simulink model "P1"  (R2023b)
settings: Solver=VariableStepAuto  StartTime=0.0  StopTime=10  RelTol=1e-3
settings Model: Creator=Usuario_UMA  LastModifiedBy=javie

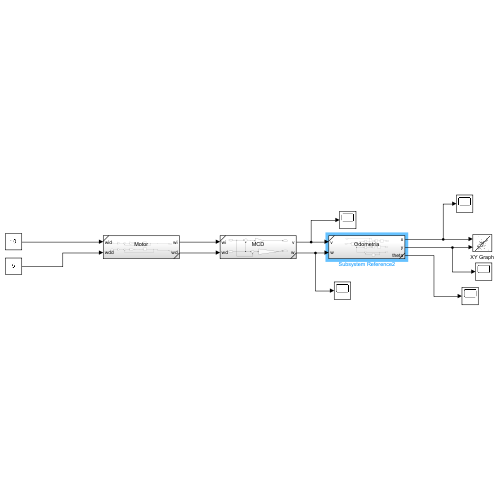
[thumbnail: Simulink's stored preview of the top-level diagram]
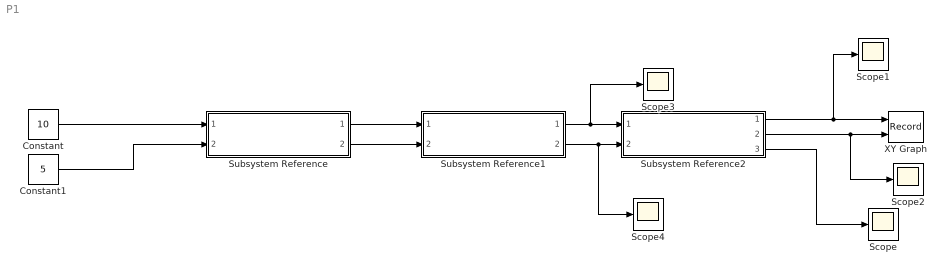
== system P1 ==
  Constant : Constant  Value=10
  Constant1 : Constant  Value=5
  Scope{,1..4} (5 alike) : Scope
  Subsystem Reference : Subsystem  ReferencedSubsystem=Motor
  Subsystem Reference1 : Subsystem  ReferencedSubsystem=MCD
  Subsystem Reference2 : Subsystem  ReferencedSubsystem=Odometria
  XY Graph : Record  FileSettingsInternal="{\"entries\":[{\"content\":{\"excelSettings\":{\"content\":{},\"type\":\"Streamout.ExcelSettings\"}},\"type\":\"Streamout.FileSettingStorage\",\"uuid\":\"\"}],\"packageUris\":[\"http:\\/\\/schema.mathworks.com\\/mf0\\/streamout_blocks\\/R2020a\"],\"version\":\"1.0\"}"  Layout=[1 1]  SignalsInternal="{\"entries\":[{\"content\":{\"signals\":[{\"content\":{\"blockPath\":[],\"dimensions\":[1],\"domain\":\"\",\"lineColor\":\"#a2142f\",\"plots\":[ 1 ],\"port\":1,\"signalID\":1,\"signalName\":\"Subsystem Reference2:1\"},\"type\":\"RecordBlkView.Signal\",\"uuid\":\"\"},{\"content\":{\"blockPath\":[],\"dimensions\":[1],\"domain\":\"\",\"lineColor\":\"#139fff\",\"plots\":[ 1 ],\"port\":2,\"signalID\":2,\"signalName\":\"Subsystem Reference2:2\"},\"type\":\"RecordBlkView.Signal\",\"uuid\":\"\"}]},\"type\":\"RecordBlkView.InputSignals\",\"uuid\":\"\"}],\"packageUris\":[\"http:\\/\\/schema.mathworks.com\\/mf0\\/streamout_blocks\\/R2020a\"],\"version\":\"1.0\"}"  VisualizationBindings="{\"xyplotplugin\":{\"info\":[{\"series\":[{\"bindingParametersList\":[{\"parameter\":\"X-Axis\",\"signalID\":1,\"signalName\":\"Subsystem Reference2:1\"},{\"parameter\":\"Y-Axis\",\"signalID\":2,\"signalName\":\"Subsystem Reference2:2\"}],\"seriesID\":0}],\"subplotID\":1}]}}"  CompatibilityTag=XY
  wires:
  Subsystem Reference/1 -> Subsystem Reference1/1
  Subsystem Reference/2 -> Subsystem Reference1/2
  Constant/1 -> Subsystem Reference/1
  Constant1/1 -> Subsystem Reference/2
  Subsystem Reference1/1 -> Scope3/1, Subsystem Reference2/1
  Subsystem Reference1/2 -> Scope4/1, Subsystem Reference2/2
  Subsystem Reference2/1 -> Scope1/1, XY Graph/1
  Subsystem Reference2/2 -> Scope2/1, XY Graph/2
  Subsystem Reference2/3 -> Scope/1
